simulink model "Delay"  (R2013a)
settings: Solver=ode45  StartTime=0.0  StopTime=10.0  RelTol=1e-3
settings Model: Creator=johanneskazantzidis  LastModifiedBy=johanneskazantzidis

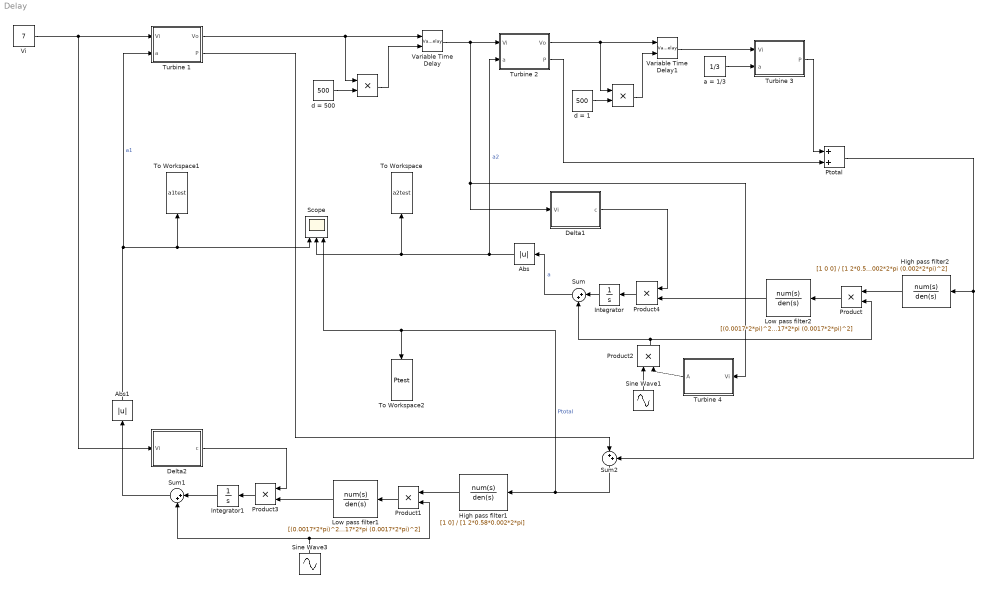
== system Delay ==
  " " : Product
  " " : Product
  Abs : Abs
  Abs1 : Abs
  Delta1 : MATLAB Function  TreatAsAtomicUnit=on
  Delta2 : MATLAB Function  TreatAsAtomicUnit=on
  High pass filter1 : TransferFcn  Numerator=[1 0]  Denominator=[1 2*0.58*0.002*2*pi]
  High pass filter2 : TransferFcn  Numerator=[1 0 0]  Denominator=[1 2*0.58*0.002*2*pi (0.002*2*pi)^2]
  Integrator : Integrator
  Integrator1 : Integrator
  Low pass filter1 : TransferFcn  Numerator=[(0.0017*2*pi)^2]  Denominator=[1 2*0.6*0.0017*2*pi (0.0017*2*pi)^2]
  Low pass filter2 : TransferFcn  Numerator=[(0.0017*2*pi)^2]  Denominator=[1 2*0.6*0.0017*2*pi (0.0017*2*pi)^2]
  Product{,1..4} (5 alike) : Product
  Ptotal : Sum
  Scope : Scope  NumInputPorts=3
      settings: ShowLegends=on  TimeRange=25000  YMin=0~0~2e+06  YMax=0.0011~0.225~2.3e+06  MaxDataPoints=200000
  Sine Wave1 : Sin  SampleTime=0
  Sine Wave3 : Sin  Amplitude=0.001  Frequency=0.95  SampleTime=0
  Sum : Sum  Inputs=|++
  Sum1 : Sum  Inputs=|++
  Sum2 : Sum  Inputs=|++
  To Workspace : ToWorkspace  VariableName=a2test  SampleTime=-1  SaveFormat=Timeseries
  To Workspace1 : ToWorkspace  VariableName=a1test  SampleTime=-1  SaveFormat=Timeseries
  To Workspace2 : ToWorkspace  VariableName=Ptest  SampleTime=-1  SaveFormat=Timeseries
  Turbine 1 : MATLAB Function  TreatAsAtomicUnit=on
  Turbine 2 : MATLAB Function  TreatAsAtomicUnit=on
  Turbine 3 : MATLAB Function  TreatAsAtomicUnit=on
  Turbine 4 : MATLAB Function  TreatAsAtomicUnit=on
  Variable Time Delay : VariableTransportDelay  MaximumDelay=10
  Variable Time Delay1 : VariableTransportDelay  MaximumDelay=10
  Vi : Constant  Value=7
  a = 1/3 : Constant  Value=1/3
  d = 1 : Constant  Value=500
  d = 500 : Constant  Value=500
  wires:
  Integrator1/1 -> Sum1/1
  Product1/1 -> Low pass filter1/1
  Low pass filter1/1 -> Product3/2
  Product3/1 -> Integrator1/1
  Delta2/1(c) -> Product3/1
  High pass filter1/1 -> Product1/1
  Turbine 1/2(P) -> Sum2/1
  Sum2/1 -> To Workspace2/1, Scope/3, High pass filter1/1  "Ptotal"
  Variable Time Delay/1 -> Turbine 2/1(Vi), Delta1/1(Vi), Turbine 4/1(Vi)
  Integrator/1 -> Sum/1
  Product4/1 -> Integrator/1
  High pass filter2/1 -> Product/1
  Sum/1 -> Abs/1  "a"
  Abs/1 -> Turbine 2/2(a), To Workspace/1, Scope/2  "a2"
  Turbine 2/2(P) -> Ptotal/2
  Turbine 3/1(P) -> Ptotal/1
  Ptotal/1 -> Sum2/2, High pass filter2/1
  a = 1/3/1 -> Turbine 3/2(a)
  Low pass filter2/1 -> Product4/2
  Product/1 -> Low pass filter2/1
  Turbine 4/1(A) -> Product2/2
  Sine Wave1/1 -> Product2/1
  Product2/1 -> Sum/2, Product/2
  Delta1/1(c) -> Product4/1
  Sum1/1 -> Abs1/1
  Abs1/1 -> Turbine 1/2(a), Scope/1, To Workspace1/1  "a1"
  Vi/1 -> Turbine 1/1(Vi), Delta2/1(Vi)
  Sine Wave3/1 -> Product1/2, Sum1/2
  Variable Time Delay1/1 -> Turbine 3/1(Vi)
  Turbine 1/1(Vo) -> " "/1, Variable Time Delay/1
  Turbine 2/1(Vo) -> " "/1, Variable Time Delay1/1
  " "/1 -> Variable Time Delay/2
  d = 500/1 -> " "/2
  d = 1/1 -> " "/2
  " "/1 -> Variable Time Delay1/2

== matlab function Delay/Turbine 1 ==
  data: Vo output; Vi input; P output; a input
function [ Vo, P] = turbineOut( Vi, a )
%turbineOut calculates a given turbine's wind speed output Vo and the
%extracted power P.
%   [Vo, P] = turbineOut(Vi,a) returns the wind speed output Vo of the 
%   given turbine and the extracted power P. Vi is the wind speed input 
%   that the turbine experiences. a is the axial induction factor.

%% Check feasability
CI = 3.5; % Cut-in speed
CO = 26; % Cut-out speed

if Vi < CI
    Vo = 0;
    P = 0;
    return
elseif  Vi > CO
    Vo = 0;
    P = 0;
    return
else
    %% Turbine specification
    R = 75;         % Blade radius m.
    rho = 1.225;    % Air density kg/m³.
    Prated = 6e6;   % Generation capability MW.
    d = 500;        % Distance in meters between this turbine and the 
                    % next. d is both the (yu-yd) and (xu-xd) which is the 
                    % distance between upstream and downstream turbines 
                    % (used for the gamma OF overlap factor.
    
    
    %% Calculate power- and wind output
    Pwind = (1/2)*rho*pi*R.^2*Vi.^3;    % Power available in the wind.
    Cp = 4*a.*(1-a).^2;                 % Power coefficient.
    P = Pwind*Cp;                       % Extracted power.
    P = min(P, Prated);                 % Limit power extraction to the 
                                        % rater power generation.
    
    
    Dc = 0.075;             % Wake-decay constant. Determined empirically.
    gammaOF = (2*R+d*Dc)/R; % Overlap factor   2R+Dcd
    Ct = 4*a.*(1-a);        % Turbine's thrust coefficient
    dV = Vi*(1-sqrt(1-Ct))*((2*R)/(2*R+2*Dc*d)).^2*gammaOF; 
                            % Velocity deficit
    
    Vo = max(Vi-dV, 0);     % Wind speed output
end

== matlab function Delay/Turbine 3 ==
  data: Vi input; P output; a input
function P  = turbineOut( Vi, a )
%UNTITLED2 Summary of this function goes here
%   Detailed explanation goes here
%% Check feasability
CI = 3.5; % Cut-in speed
CO = 26; % Cut-out speed

if Vi < CI
    Vo = 0;
    P = 0;
    return
elseif  Vi > CO
    Vo = 0;
    P = 0;
    return
else
    %% Declarations
    R = 75; % Blade radius m
    rho = 1.225; % Air density kg/m³
    Prated = 6e6; % Generation capability MW
    d = 500; % Distance in m between this turbine and the next. d is both the
    % (yu-yd) and (xu-xd) which is the distance between upstream and
    % downstream turbines (used for the gamma OF overlap factor
    
    
    %% Calculate power
    % Note that wind output is irrelevant since this is the last turbine.
    Pwind = (1/2)*rho*pi*R.^2*Vi.^3;
    Cp = 4*a.*(1-a).^2;
    P = Pwind*Cp; 
    P = min(P, Prated);
    
    Dc = 0.075; % Wake-decay constant. Determined empirically;
    gammaOF = (2*R+d*Dc)/R; % Overlap factor   2R+Dcd
    Ct = 4*a.*(1-a); % Turbine's thrust coefficient
    dV = Vi*(1-sqrt(1-Ct))*((2*R)/(2*R+2*Dc*d)).^2*gammaOF; % Velocity deficit
    
    Vo = max(Vi-dV, 0);
end

== matlab function Delay/Turbine 4 ==
  data: A output; Vi input
% function A = Amplitude( Vi )
% %UNTITLED2 Summary of this function goes here
% %   Detailed explanation goes here
% if Vi<=7.5
%     A = 4e-3;
% elseif Vi>12.5
%     A = 4.5e-3;
% elseif Vi>11.5 && Vi<=12.5
%     A = 4e-3;
% elseif Vi>10.5 && Vi<=11.5
%     A = 7e-3;
% elseif Vi>8.5 && Vi<=10.5
%     A = 5e-3;
% else
%     A = 6e-3;
% end
% end

function A = Amplitude( Vi )
%UNTITLED2 Summary of this function goes here
%   Detailed explanation goes here
if Vi<=7.5
    %A = 5.5e-3;
    A = 4e-3;
elseif Vi>12.5
    A = 4.5e-3;
elseif Vi>11.5 && Vi<=12.5
    A = 4e-3;
elseif Vi>10.5 && Vi<=11.5
    A = 7e-3;
elseif Vi>8.5 && Vi<=10.5
    A = 5e-3;
else
    A = 6e-3;
end
end

== matlab function Delay/Delta1 ==
  data: c output; Vi input
% function c   = delta( Vi )
% %UNTITLED2 Summary of this function goes here
% %   Detailed explanation goes here
% if Vi<=7.5
%     c = 8e-5;
% elseif Vi>=12.5
%     c = 3e-7;
% elseif Vi>=9.5 && Vi<10.5
%     c = 5e-6;
% elseif Vi>=10.5 && Vi<12.5
%     c = 1e-7;
% else
%     c = 8e-6;
% end
% end



function c   = delta( Vi )
%UNTITLED2 Summary of this function goes here
%   Detailed explanation goes here
if Vi<=7.5
    %c = 1.5e-6;
    c = 5e-6;
elseif Vi>=12.5
    c = 3e-7;
elseif Vi>=9.5 && Vi<10.5
    c = 5e-6;
elseif Vi>=10.5 && Vi<12.5
    c = 1e-7;
else
    c = 8e-6;
end
end

== matlab function Delay/Turbine 2 ==
  data: Vo output; Vi input; P output; a input
function [ Vo, P] = turbineOut( Vi, a )
%UNTITLED2 Summary of this function goes here
%   Detailed explanation goes here
%% Check feasability
CI = 3.5; % Cut-in speed
CO = 26; % Cut-out speed

if Vi < CI
    Vo = 0;
    P = 0;
    return
elseif  Vi > CO
    Vo = 0;
    P = 0;
    return
else
    %% Declarations
    R = 75; % Blade radius m
    rho = 1.225; % Air density kg/m³
    Prated = 6e6; % Generation capability MW
    d = 500; % Distance in m between this turbine and the next. d is both the
    % (yu-yd) and (xu-xd) which is the distance between upstream and
    % downstream turbines (used for the gamma OF overlap factor
    
    
    %% Calculate power- and wind output
    Pwind = (1/2)*rho*pi*R.^2*Vi.^3;
    Cp = 4*a.*(1-a).^2;
    P = Pwind*Cp;
    P = min(P, Prated);
    
    
    Dc = 0.075; % Wake-decay constant. Determined empirically;
    gammaOF = (2*R+d*Dc)/R; % Overlap factor   2R+Dcd
    Ct = 4*a.*(1-a); % Turbine's thrust coefficient
    dV = Vi*(1-sqrt(1-Ct))*((2*R)/(2*R+2*Dc*d)).^2*gammaOF; % Velocity deficit
    
    Vo = max(Vi-dV, 0);
end

== matlab function Delay/Delta2 ==
  data: c output; Vi input
function c   = delta( Vi )
%UNTITLED2 Summary of this function goes here
%   Detailed explanation goes here
if Vi<=7.5 %perhaps 6.5?
    c = 2e-8;
%elseif Vi>6.5 && Vi<=7.5
 %   c = 2e-7;
elseif Vi>7.5 && Vi<9.5
    c = 8e-8;
elseif Vi>=9.5 && Vi<10.5
    c = 2e-8;
elseif Vi>=10.5 && Vi<11.5
    %c = 8e-10;
 c = 4e-6;
    
elseif Vi>=11.5 && Vi<12.5
    c = 7.6e-6;
else
    c = 1e-6;
end
end
